simulink model "a7_"  (R2023b)
settings: Solver=ode45  StartTime=0.0  StopTime=40.0  MaxStep=0.01  RelTol=1e-3  EnableMultiTasking=on
settings Model: Creator=andre.bergmann  LastModifiedBy=LUCAS
settings SolverCC: AlgebraicLoopSolver=TrustRegion
settings DataIOCC: LimitDataPoints=on  SaveFormat=Array  ReturnWorkspaceOutputs=off
settings OptimizationCC: ExpressionDepthLimit=2147483647  LifeSpan=inf
settings DebuggingCC: UnderspecifiedInitializationDetection=Classic  MergeDetectMultiDrivingBlocksExec=none  SolverPrmCheckMsg=warning  UnconnectedInputMsg=warning  UnconnectedOutputMsg=warning  UnconnectedLineMsg=warning  StateNameClashWarn=warning  SFUnexpectedBacktrackingDiag=warning  SFNoUnconditionalDefaultTransitionDiag=warning  SFExecutionAtInitializationDiag=none  ArithmeticOperatorsInVariantConditions=warning
settings HardwareCC: ProdBitPerPointer=32  ProdBitPerSizeT=32  ProdBitPerPtrDiffT=32  ProdLargestAtomicFloat=None  ProdIntDivRoundTo=Undefined  ProdEndianess=Unspecified  ProdWordSize=32  ProdHWDeviceType=32-bit Generic
settings ModelReferenceCC: PropagateSignalLabelsOutOfModel=off
settings SFSimCC: SimUseLocalCustomCode=off  CustomCodeUndefinedFunction=UseInterfaceOnly
settings RTWCC: RTWUseLocalCustomCode=off
settings CodeAppCC: StateflowObjectComments=on
settings GRTTargetCC: TargetLangStandard=C89/C90 (ANSI)
settings ConfigComp: CovMetricSettings=dw  CovSaveCumulativeToWorkspaceVar=on  CovSaveSingleToWorkspaceVar=on  CovExternalEMLEnable=off

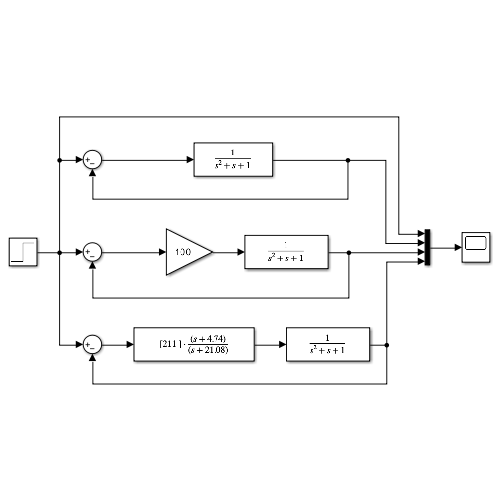
[thumbnail: Simulink's stored preview of the top-level diagram]
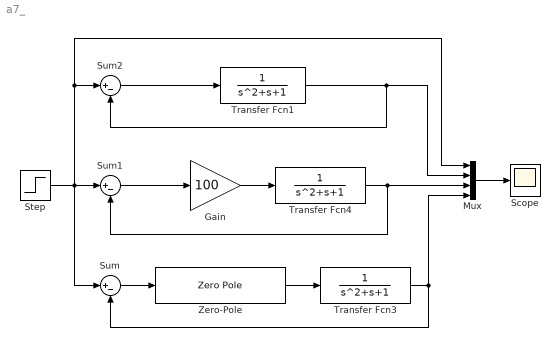
== system a7_ ==
  Gain : Gain  Gain=100
  Mux : Mux
  Scope : Scope
  Step : Step  SampleTime=0
  Sum : Sum  Inputs=|+-
  Sum1 : Sum  Inputs=|+-
  Sum2 : Sum  Inputs=|+-
  Transfer Fcn1 : TransferFcn  Denominator=[1 1 1]
  Transfer Fcn3 : TransferFcn  Denominator=[1 1 1]
  Transfer Fcn4 : TransferFcn  Denominator=[1 1 1]
  Zero-Pole : ZeroPole  Zeros=[-4.74]  Poles=[-21.08]  Gain=[211]
  wires:
  Step/1 -> Mux/1, Sum2/1, Sum/1, Sum1/1
  Sum2/1 -> Transfer Fcn1/1
  Transfer Fcn1/1 -> Mux/2, Sum2/2
  Sum1/1 -> Gain/1
  Gain/1 -> Transfer Fcn4/1
  Transfer Fcn4/1 -> Sum1/2, Mux/3
  Transfer Fcn3/1 -> Mux/4, Sum/2
  Zero-Pole/1 -> Transfer Fcn3/1
  Sum/1 -> Zero-Pole/1
  Mux/1 -> Scope/1
